simulink model "KUKA_Linear"  (R2020b)
settings: Solver=VariableStepAuto  StartTime=0.0  StopTime=200  RelTol=1e-3
(part 2 of 3)

== matlab function KUKA_Linear/ 4DoF KUKA LWR4+ Dynamics ==
  data: q input; q_dot input; torque input; q_ddot output
function q_ddot = fcn(q,q_dot,torque)
%#codegen

%% parameters
td1 = q_dot(1);
td2 = q_dot(2);
td3 = q_dot(3);
td4 = q_dot(4);

%% Constant

d3 = 0.4;

m1 = 2.7;
m2 = 2.7;
m3 = 2.7;
m4 = 2.7;

cx1 = 0.001340;
cx2 = 0.001340;
cx3 = -0.001340;
cx4 = -0.001340;

cy1 = -0.87777;
cy2 = -0.02622;
cy3 = 0.87777;
cy4 = 0.02622;

cz1 = -0.02622;
cz2 = 0.87777;
cz3 = -0.02622;
cz4 = 0.87777;

g = 9.8;

Ixx1 = 0.039; 
Ixy1 = 3.206e-4;
Ixz1 = 9.415e-5;
Iyy1 = 6.887e-3;
Iyz1 = -2.681e-3;
Izz1 = 0.03698;

Ixx2 = 0.039; 
Ixy2 = 9.415e-5;
Ixz2 = -3.145e-4;
Iyy2 = 0.03698;
Iyz2 = 9.747e-3;
Izz2 = 6.887e-3;

Ixx3 = 6.887e-3; 
Ixy3 = 3.145e-4;
Ixz3 = -9.5572e-5;
Iyy3 = 6.8872e-3;
Iyz3 = 2.681e-3;
Izz3 = 0.037;

Ixx4 = 0.037; 
Ixy4 = 9.415e-5;
Ixz4 = 3.1455e-4;
Iyy4 = 0.037;
Iyz4 = 9.747e-3;
Izz4 = 6.887e-3;

%% Triangle relative
c1 = cos(q(1));
c2 = cos(q(2));
c3 = cos(q(3));
c4 = cos(q(4)); 

s1 = sin(q(1));
s2 = sin(q(2));
s3 = sin(q(3));
s4 = sin(q(4));

%% matrix M

m11 = m1*cx1^2 + m1*cy1^2 + Izz1 - Iyz2*c2 - Ixz2*s2 - s2*(Ixz3*c2 + c3*(Ixx4*(c2*s4 - c3*c4*s2) - Ixy4*(c2*c4 + c3*s2*s4) + cy4*m4*(cy4*(c2*s4 - c3*c4*s2) - cx4*(c2*c4 + c3*s2*s4) + c3*d3*s2) + cz4*m4*(cz4*(c2*s4 - c3*c4*s2) - cx4*s2*s3 + d3*s2*s3*s4) - Ixz4*s2*s3) + s3*(Ixy4*(c2*s4 - c3*c4*s2) - Iyy4*(c2*c4 + c3*s2*s4) + cx4*m4*(cy4*(c2*s4 - c3*c4*s2) - cx4*(c2*c4 + c3*s2*s4) + c3*d3*s2) - cz4*m4*(cz4*(c2*c4 + c3*s2*s4) - cy4*s2*s3 + c4*d3*s2*s3) + Iyz4*s2*s3) - d3*m4*(cy4*(c2*s4 - c3*c4*s2) - cx4*(c2*c4 + c3*s2*s4) + c3*d3*s2) + cz3*m3*(c2*cx3 - c3*cz3*s2) - Ixx3*c3*s2 - Ixy3*s2*s3 - cy3*m3*(c3*cy3*s2 + cx3*s2*s3)) - c2*(Iyz3*c2 + d3*(c3*m4*(cz4*(c2*c4 + c3*s2*s4) - cy4*s2*s3 + c4*d3*s2*s3) + m4*s3*(cz4*(c2*s4 - c3*c4*s2) - cx4*s2*s3 + d3*s2*s3*s4)) - Ixz4*(c2*s4 - c3*c4*s2) - Iyz4*(c2*c4 + c3*s2*s4) - cy4*m4*(cz4*(c2*c4 + c3*s2*s4) - cy4*s2*s3 + c4*d3*s2*s3) - cx4*m4*(cz4*(c2*s4 - c3*c4*s2) - cx4*s2*s3 + d3*s2*s3*s4) + cz3*m3*(c2*cy3 + cz3*s2*s3) + Ixy3*c3*s2 + Iyy3*s2*s3 + Izz4*s2*s3 + cx3*m3*(c3*cy3*s2 + cx3*s2*s3)) - cx2*cz2*m2*s2 - c2*cy2*cz2*m2;
m12 = m2*cx2^2 + m2*cy2^2 + Izz2 - c2*(c3*m3*cz3^2 - d3*(c3*m4*(c3*cy4 - c3*c4*d3 + cz4*s3*s4) - m4*s3*(c4*cz4*s3 - c3*cx4 + c3*d3*s4)) + Iyy3*c3 + Izz4*c3 - Ixy3*s3 - Ixz4*c4*s3 + Iyz4*s3*s4 - cx4*m4*(c4*cz4*s3 - c3*cx4 + c3*d3*s4) + cy4*m4*(c3*cy4 - c3*c4*d3 + cz4*s3*s4) + cx3*m3*(c3*cx3 - cy3*s3)) - s2*(m3*s3*cz3^2 - Ixy3*c3 + Ixx3*s3 + c3*(cy4*m4*(c4*cy4*s3 - d3*s3 + cx4*s3*s4) - Ixz4*c3 + Ixx4*c4*s3 + Ixy4*s3*s4 + cz4*m4*(c4*cz4*s3 - c3*cx4 + c3*d3*s4)) + s3*(Iyz4*c3 + cx4*m4*(c4*cy4*s3 - d3*s3 + cx4*s3*s4) + Ixy4*c4*s3 + Iyy4*s3*s4 + cz4*m4*(c3*cy4 - c3*c4*d3 + cz4*s3*s4)) - d3*m4*(c4*cy4*s3 - d3*s3 + cx4*s3*s4) - cy3*m3*(c3*cx3 - cy3*s3));
m13 = c2*(Iyz4*c4 - Iyz3 + Ixz4*s4 - d3*(cz4*m4*s3*s4 + c3*c4*cz4*m4) - cy3*cz3*m3 + cx4*cz4*m4*s4 + c4*cy4*cz4*m4) - s2*(Ixz3 - c3*(- m4*s4*cz4^2 + Ixy4*c4 - Ixx4*s4 + cy4*m4*(c4*cx4 - cy4*s4)) - s3*(c4*m4*cz4^2 + Iyy4*c4 - Ixy4*s4 + cx4*m4*(c4*cx4 - cy4*s4)) + cx3*cz3*m3 + d3*m4*(c4*cx4 - cy4*s4));
m14 = s2*(s3*(Iyz4 + cy4*cz4*m4) - c3*(Ixz4 + cx4*cz4*m4)) + c2*(Izz4 - d3*(c3*cy4*m4 + cx4*m4*s3) + cx4^2*m4 + cy4^2*m4);

m21 = - Iyz2*c2 - Ixz2*s2 - s2*(Ixz3*c2 + c3*(Ixx4*(c2*s4 - c3*c4*s2) - Ixy4*(c2*c4 + c3*s2*s4) + cy4*m4*(cy4*(c2*s4 - c3*c4*s2) - cx4*(c2*c4 + c3*s2*s4) + c3*d3*s2) + cz4*m4*(cz4*(c2*s4 - c3*c4*s2) - cx4*s2*s3 + d3*s2*s3*s4) - Ixz4*s2*s3) + s3*(Ixy4*(c2*s4 - c3*c4*s2) - Iyy4*(c2*c4 + c3*s2*s4) + cx4*m4*(cy4*(c2*s4 - c3*c4*s2) - cx4*(c2*c4 + c3*s2*s4) + c3*d3*s2) - cz4*m4*(cz4*(c2*c4 + c3*s2*s4) - cy4*s2*s3 + c4*d3*s2*s3) + Iyz4*s2*s3) - d3*m4*(cy4*(c2*s4 - c3*c4*s2) - cx4*(c2*c4 + c3*s2*s4) + c3*d3*s2) + cz3*m3*(c2*cx3 - c3*cz3*s2) - Ixx3*c3*s2 - Ixy3*s2*s3 - cy3*m3*(c3*cy3*s2 + cx3*s2*s3)) - c2*(Iyz3*c2 + d3*(c3*m4*(cz4*(c2*c4 + c3*s2*s4) - cy4*s2*s3 + c4*d3*s2*s3) + m4*s3*(cz4*(c2*s4 - c3*c4*s2) - cx4*s2*s3 + d3*s2*s3*s4)) - Ixz4*(c2*s4 - c3*c4*s2) - Iyz4*(c2*c4 + c3*s2*s4) - cy4*m4*(cz4*(c2*c4 + c3*s2*s4) - cy4*s2*s3 + c4*d3*s2*s3) - cx4*m4*(cz4*(c2*s4 - c3*c4*s2) - cx4*s2*s3 + d3*s2*s3*s4) + cz3*m3*(c2*cy3 + cz3*s2*s3) + Ixy3*c3*s2 + Iyy3*s2*s3 + Izz4*s2*s3 + cx3*m3*(c3*cy3*s2 + cx3*s2*s3)) - cx2*cz2*m2*s2 - c2*cy2*cz2*m2;
m22 = m2*cx2^2 + m2*cy2^2 + Izz2 - c2*(c3*m3*cz3^2 - d3*(c3*m4*(c3*cy4 - c3*c4*d3 + cz4*s3*s4) - m4*s3*(c4*cz4*s3 - c3*cx4 + c3*d3*s4)) + Iyy3*c3 + Izz4*c3 - Ixy3*s3 - Ixz4*c4*s3 + Iyz4*s3*s4 - cx4*m4*(c4*cz4*s3 - c3*cx4 + c3*d3*s4) + cy4*m4*(c3*cy4 - c3*c4*d3 + cz4*s3*s4) + cx3*m3*(c3*cx3 - cy3*s3)) - s2*(m3*s3*cz3^2 - Ixy3*c3 + Ixx3*s3 + c3*(cy4*m4*(c4*cy4*s3 - d3*s3 + cx4*s3*s4) - Ixz4*c3 + Ixx4*c4*s3 + Ixy4*s3*s4 + cz4*m4*(c4*cz4*s3 - c3*cx4 + c3*d3*s4)) + s3*(Iyz4*c3 + cx4*m4*(c4*cy4*s3 - d3*s3 + cx4*s3*s4) + Ixy4*c4*s3 + Iyy4*s3*s4 + cz4*m4*(c3*cy4 - c3*c4*d3 + cz4*s3*s4)) - d3*m4*(c4*cy4*s3 - d3*s3 + cx4*s3*s4) - cy3*m3*(c3*cx3 - cy3*s3));
m23 = c2*(Iyz4*c4 - Iyz3 + Ixz4*s4 - d3*(cz4*m4*s3*s4 + c3*c4*cz4*m4) - cy3*cz3*m3 + cx4*cz4*m4*s4 + c4*cy4*cz4*m4) - s2*(Ixz3 - c3*(- m4*s4*cz4^2 + Ixy4*c4 - Ixx4*s4 + cy4*m4*(c4*cx4 - cy4*s4)) - s3*(c4*m4*cz4^2 + Iyy4*c4 - Ixy4*s4 + cx4*m4*(c4*cx4 - cy4*s4)) + cx3*cz3*m3 + d3*m4*(c4*cx4 - cy4*s4));
m24 = s2*(s3*(Iyz4 + cy4*cz4*m4) - c3*(Ixz4 + cx4*cz4*m4)) + c2*(Izz4 - d3*(c3*cy4*m4 + cx4*m4*s3) + cx4^2*m4 + cy4^2*m4);

m31 = Izz3*c2 - c3*(Ixy4*(c2*s4 - c3*c4*s2) - Iyy4*(c2*c4 + c3*s2*s4) + cx4*m4*(cy4*(c2*s4 - c3*c4*s2) - cx4*(c2*c4 + c3*s2*s4) + c3*d3*s2) - cz4*m4*(cz4*(c2*c4 + c3*s2*s4) - cy4*s2*s3 + c4*d3*s2*s3) + Iyz4*s2*s3) + s3*(Ixx4*(c2*s4 - c3*c4*s2) - Ixy4*(c2*c4 + c3*s2*s4) + cy4*m4*(cy4*(c2*s4 - c3*c4*s2) - cx4*(c2*c4 + c3*s2*s4) + c3*d3*s2) + cz4*m4*(cz4*(c2*s4 - c3*c4*s2) - cx4*s2*s3 + d3*s2*s3*s4) - Ixz4*s2*s3) + cx3*m3*(c2*cx3 - c3*cz3*s2) + cy3*m3*(c2*cy3 + cz3*s2*s3) - Ixz3*c3*s2 + Iyz3*s2*s3;
m32 = Iyz3*c3 + Ixz3*s3 - c3*(Iyz4*c3 + cx4*m4*(c4*cy4*s3 - d3*s3 + cx4*s3*s4) + Ixy4*c4*s3 + Iyy4*s3*s4 + cz4*m4*(c3*cy4 - c3*c4*d3 + cz4*s3*s4)) + s3*(cy4*m4*(c4*cy4*s3 - d3*s3 + cx4*s3*s4) - Ixz4*c3 + Ixx4*c4*s3 + Ixy4*s3*s4 + cz4*m4*(c4*cz4*s3 - c3*cx4 + c3*d3*s4)) + cx3*cz3*m3*s3 + c3*cy3*cz3*m3;
m33 = m3*cx3^2 + m3*cy3^2 + Izz3 + c3*(c4*m4*cz4^2 + Iyy4*c4 - Ixy4*s4 + cx4*m4*(c4*cx4 - cy4*s4)) - s3*(- m4*s4*cz4^2 + Ixy4*c4 - Ixx4*s4 + cy4*m4*(c4*cx4 - cy4*s4));
m34 = s3*(Ixz4 + cx4*cz4*m4) + c3*(Iyz4 + cy4*cz4*m4);

m41 = Ixz4*(c2*s4 - c3*c4*s2) + Iyz4*(c2*c4 + c3*s2*s4) + cy4*m4*(cz4*(c2*c4 + c3*s2*s4) - cy4*s2*s3 + c4*d3*s2*s3) + cx4*m4*(cz4*(c2*s4 - c3*c4*s2) - cx4*s2*s3 + d3*s2*s3*s4) - Izz4*s2*s3;
m42 = Ixz4*c4*s3 - Izz4*c3 - Iyz4*s3*s4 + cx4*m4*(c4*cz4*s3 - c3*cx4 + c3*d3*s4) - cy4*m4*(c3*cy4 - c3*c4*d3 + cz4*s3*s4);
m43 = Iyz4*c4 + Ixz4*s4 + cx4*cz4*m4*s4 + c4*cy4*cz4*m4;
m44 = m4*cx4^2 + m4*cy4^2 + Izz4;

M = [m11 m12 m13 m14;
     m21 m22 m23 m24;
     m31 m32 m33 m34;
     m41 m42 m43 m44];
 
%% matrix V

corio1 = (td2^2*(c2*(2*s3*(Iyz3*c3 + Ixz3*s3) - d3*(c3*m4*(2*c3*(c3*cx4 - c4*cz4*s3) - s4*(2*d3*c3^2 + 2*d3*s3^2) + 2*s3*s4*(c4*cy4*s3 + cx4*s3*s4)) - m4*s3*(2*c3*(c3*cy4 + cz4*s3*s4) - c4*(2*d3*c3^2 + 2*d3*s3^2) + 2*c4*s3*(c4*cy4*s3 + cx4*s3*s4))) - cx4*m4*(2*c3*(c3*cy4 + cz4*s3*s4) - c4*(2*d3*c3^2 + 2*d3*s3^2) + 2*c4*s3*(c4*cy4*s3 + cx4*s3*s4)) + cy4*m4*(2*c3*(c3*cx4 - c4*cz4*s3) - s4*(2*d3*c3^2 + 2*d3*s3^2) + 2*s3*s4*(c4*cy4*s3 + cx4*s3*s4)) + cx3*m3*(2*cz3*c3^2 + 2*cz3*s3^2) - 2*c4*s3*(Iyz4*c3 + Ixy4*c4*s3 + Iyy4*s3*s4) + 2*s3*s4*(Ixx4*c4*s3 - Ixz4*c3 + Ixy4*s3*s4) - 2*c3*cz3*m3*(c3*cx3 - cy3*s3)) - s2*(2*c3*(Iyz3*c3 + Ixz3*s3) - s3*(cx4*m4*(2*c4*s3*(c3*cx4 - c4*cz4*s3) - 2*s3*s4*(c3*cy4 + cz4*s3*s4)) - 2*c3*(Ixx4*c4*s3 - Ixz4*c3 + Ixy4*s3*s4) + cz4*m4*(2*c3*(c3*cx4 - c4*cz4*s3) - s4*(2*d3*c3^2 + 2*d3*s3^2) + 2*s3*s4*(c4*cy4*s3 + cx4*s3*s4)) + 2*c4*s3*(Izz4*c3 - Ixz4*c4*s3 + Iyz4*s3*s4)) - c3*(2*c3*(Iyz4*c3 + Ixy4*c4*s3 + Iyy4*s3*s4) + cy4*m4*(2*c4*s3*(c3*cx4 - c4*cz4*s3) - 2*s3*s4*(c3*cy4 + cz4*s3*s4)) + cz4*m4*(2*c3*(c3*cy4 + cz4*s3*s4) - c4*(2*d3*c3^2 + 2*d3*s3^2) + 2*c4*s3*(c4*cy4*s3 + cx4*s3*s4)) - 2*s3*s4*(Izz4*c3 - Ixz4*c4*s3 + Iyz4*s3*s4)) + d3*m4*(2*c4*s3*(c3*cx4 - c4*cz4*s3) - 2*s3*s4*(c3*cy4 + cz4*s3*s4)) + cy3*m3*(2*cz3*c3^2 + 2*cz3*s3^2) + 2*cz3*m3*s3*(c3*cx3 - cy3*s3))))/2 + (td3^2*(s2*(2*Iyz3 - c3*(2*c4*(Iyz4*c4 + Ixz4*s4) + cy4*m4*(2*cz4*c4^2 + 2*cz4*s4^2) + 2*cz4*m4*s4*(c4*cx4 - cy4*s4)) - s3*(2*s4*(Iyz4*c4 + Ixz4*s4) + cx4*m4*(2*cz4*c4^2 + 2*cz4*s4^2) - 2*c4*cz4*m4*(c4*cx4 - cy4*s4)) + 2*cy3*cz3*m3 + d3*m4*(2*cz4*c4^2 + 2*cz4*s4^2)) + c2*(2*c4*(Ixy4*c4 - Ixx4*s4) - 2*Ixz3 + 2*s4*(Iyy4*c4 - Ixy4*s4) - d3*(2*c3*c4*m4*(c4*cx4 - cy4*s4) + 2*m4*s3*s4*(c4*cx4 - cy4*s4)) - 2*cx3*cz3*m3 + 2*c4*cy4*m4*(c4*cx4 - cy4*s4) + 2*cx4*m4*s4*(c4*cx4 - cy4*s4))))/2 + (td4^2*(s2*(c3*(2*Iyz4 + 2*cy4*cz4*m4) + s3*(2*Ixz4 + 2*cx4*cz4*m4)) - c2*d3*(2*c3*cx4*m4 - 2*cy4*m4*s3)))/2 + (td1^2*(s2*(2*c2*(Iyz3*c2 + Ixy3*c3*s2 + Iyy3*s2*s3) - c3*(2*(c2*c4 + c3*s2*s4)*(Ixz4*(c2*s4 - c3*c4*s2) + Iyz4*(c2*c4 + c3*s2*s4) - Izz4*s2*s3) + cy4*m4*(2*(c2*s4 - c3*c4*s2)*(cz4*(c2*s4 - c3*c4*s2) - cx4*s2*s3) + 2*(c2*c4 + c3*s2*s4)*(cz4*(c2*c4 + c3*s2*s4) - cy4*s2*s3) + 2*c2*d3*s2*s3) - 2*s2*s3*(Ixy4*(c2*s4 - c3*c4*s2) - Iyy4*(c2*c4 + c3*s2*s4) + Iyz4*s2*s3) + cz4*m4*(2*(c2*s4 - c3*c4*s2)*(cx4*(c2*c4 + c3*s2*s4) - cy4*(c2*s4 - c3*c4*s2)) + c4*(2*d3*c3^2*s2^2 + 2*d3*s2^2*s3^2) + 2*s2*s3*(cz4*(c2*c4 + c3*s2*s4) - cy4*s2*s3) - 2*c2*c3*d3*s2*s4)) - s3*(2*(c2*s4 - c3*c4*s2)*(Ixz4*(c2*s4 - c3*c4*s2) + Iyz4*(c2*c4 + c3*s2*s4) - Izz4*s2*s3) + cx4*m4*(2*(c2*s4 - c3*c4*s2)*(cz4*(c2*s4 - c3*c4*s2) - cx4*s2*s3) + 2*(c2*c4 + c3*s2*s4)*(cz4*(c2*c4 + c3*s2*s4) - cy4*s2*s3) + 2*c2*d3*s2*s3) - 2*s2*s3*(Ixy4*(c2*c4 + c3*s2*s4) - Ixx4*(c2*s4 - c3*c4*s2) + Ixz4*s2*s3) + cz4*m4*(s4*(2*d3*c3^2*s2^2 + 2*d3*s2^2*s3^2) - 2*(c2*c4 + c3*s2*s4)*(cx4*(c2*c4 + c3*s2*s4) - cy4*(c2*s4 - c3*c4*s2)) + 2*s2*s3*(cz4*(c2*s4 - c3*c4*s2) - cx4*s2*s3) + 2*c2*c3*c4*d3*s2)) + cz3*m3*(2*c2*(c2*cy3 + cz3*s2*s3) + 2*c3*s2*(c3*cy3*s2 + cx3*s2*s3)) + cy3*m3*(2*c3*s2*(c2*cx3 - c3*cz3*s2) - 2*s2*s3*(c2*cy3 + cz3*s2*s3)) + d3*m4*(2*(c2*s4 - c3*c4*s2)*(cz4*(c2*s4 - c3*c4*s2) - cx4*s2*s3) + 2*(c2*c4 + c3*s2*s4)*(cz4*(c2*c4 + c3*s2*s4) - cy4*s2*s3) + 2*c2*d3*s2*s3) - 2*s2*s3*(Izz3*c2 - Ixz3*c3*s2 + Iyz3*s2*s3)) + 2*c2*(Ixy2*c2 - Ixx2*s2) + 2*s2*(Iyy2*c2 - Ixy2*s2) - c2*(2*(c2*s4 - c3*c4*s2)*(Ixy4*(c2*s4 - c3*c4*s2) - Iyy4*(c2*c4 + c3*s2*s4) + Iyz4*s2*s3) - 2*(c2*c4 + c3*s2*s4)*(Ixy4*(c2*c4 + c3*s2*s4) - Ixx4*(c2*s4 - c3*c4*s2) + Ixz4*s2*s3) - d3*(c3*m4*(s4*(2*d3*c3^2*s2^2 + 2*d3*s2^2*s3^2) - 2*(c2*c4 + c3*s2*s4)*(cx4*(c2*c4 + c3*s2*s4) - cy4*(c2*s4 - c3*c4*s2)) + 2*s2*s3*(cz4*(c2*s4 - c3*c4*s2) - cx4*s2*s3) + 2*c2*c3*c4*d3*s2) - m4*s3*(2*(c2*s4 - c3*c4*s2)*(cx4*(c2*c4 + c3*s2*s4) - cy4*(c2*s4 - c3*c4*s2)) + c4*(2*d3*c3^2*s2^2 + 2*d3*s2^2*s3^2) + 2*s2*s3*(cz4*(c2*c4 + c3*s2*s4) - cy4*s2*s3) - 2*c2*c3*d3*s2*s4)) - 2*c2*(Ixx3*c3*s2 - Ixz3*c2 + Ixy3*s2*s3) + cx3*m3*(2*c3*s2*(c2*cx3 - c3*cz3*s2) - 2*s2*s3*(c2*cy3 + cz3*s2*s3)) + cz3*m3*(2*c2*(c2*cx3 - c3*cz3*s2) + 2*s2*s3*(c3*cy3*s2 + cx3*s2*s3)) + 2*c3*s2*(Izz3*c2 - Ixz3*c3*s2 + Iyz3*s2*s3) - cx4*m4*(2*(c2*s4 - c3*c4*s2)*(cx4*(c2*c4 + c3*s2*s4) - cy4*(c2*s4 - c3*c4*s2)) + c4*(2*d3*c3^2*s2^2 + 2*d3*s2^2*s3^2) + 2*s2*s3*(cz4*(c2*c4 + c3*s2*s4) - cy4*s2*s3) - 2*c2*c3*d3*s2*s4) + cy4*m4*(s4*(2*d3*c3^2*s2^2 + 2*d3*s2^2*s3^2) - 2*(c2*c4 + c3*s2*s4)*(cx4*(c2*c4 + c3*s2*s4) - cy4*(c2*s4 - c3*c4*s2)) + 2*s2*s3*(cz4*(c2*s4 - c3*c4*s2) - cx4*s2*s3) + 2*c2*c3*c4*d3*s2)) + 2*c2*cy2*m2*(c2*cx2 - cy2*s2) + 2*cx2*m2*s2*(c2*cx2 - cy2*s2)))/2 - td2*td4*(s2*(s3*(2*Ixz4*c3 - Ixx4*c4*s3 + Iyy4*c4*s3 + Izz4*c4*s3 - 2*Ixy4*s3*s4 + cx4*m4*(2*c4*cx4*s3 - 2*cy4*s3*s4) + 2*c3*cx4*cz4*m4) + c3*(2*Iyz4*c3 + 2*Ixy4*c4*s3 - Ixx4*s3*s4 + Iyy4*s3*s4 - Izz4*s3*s4 + cy4*m4*(2*c4*cx4*s3 - 2*cy4*s3*s4) + 2*c3*cy4*cz4*m4) - d3*m4*(2*c4*cx4*s3 - 2*cy4*s3*s4)) - c2*d3*(2*c3^2*cx4*m4 - 2*c3*cy4*m4*s3)) - td1*td3*(c2*(2*Ixz3*c2 - (c2*c4 + c3*s2*s4)*(Ixy4*c4 - Ixx4*s4) - (c2*s4 - c3*c4*s2)*(Iyy4*c4 - Ixy4*s4) + d3*(c3*m4*(c4*(cx4*(c2*c4 + c3*s2*s4) - cy4*(c2*s4 - c3*c4*s2)) + (c2*c4 + c3*s2*s4)*(c4*cx4 - cy4*s4) - c3*cy4*s2 - 2*cz4*s2*s3*s4) + m4*s3*(s4*(cx4*(c2*c4 + c3*s2*s4) - cy4*(c2*s4 - c3*c4*s2)) + (c2*s4 - c3*c4*s2)*(c4*cx4 - cy4*s4) - c3*cx4*s2 + 2*c4*cz4*s2*s3)) - c4*(Ixy4*(c2*c4 + c3*s2*s4) - Ixx4*(c2*s4 - c3*c4*s2) + Ixz4*s2*s3) + s4*(Ixy4*(c2*s4 - c3*c4*s2) - Iyy4*(c2*c4 + c3*s2*s4) + Iyz4*s2*s3) - Ixx3*c3*s2 + Iyy3*c3*s2 + Izz3*c3*s2 + Izz4*c3*s2 - cx4*m4*(s4*(cx4*(c2*c4 + c3*s2*s4) - cy4*(c2*s4 - c3*c4*s2)) + (c2*s4 - c3*c4*s2)*(c4*cx4 - cy4*s4) - c3*cx4*s2 + 2*c4*cz4*s2*s3) - cy4*m4*(c4*(cx4*(c2*c4 + c3*s2*s4) - cy4*(c2*s4 - c3*c4*s2)) + (c2*c4 + c3*s2*s4)*(c4*cx4 - cy4*s4) - c3*cy4*s2 - 2*cz4*s2*s3*s4) - 2*Ixy3*s2*s3 + cx3*m3*(2*c3*cx3*s2 - 2*cy3*s2*s3) + Iyz4*s2*s3*s4 - Ixz4*c4*s2*s3 + 2*c2*cx3*cz3*m3) - s2*(2*Iyz3*c2 - c3*((c2*c4 + c3*s2*s4)*(Iyz4*c4 + Ixz4*s4) + c4*(Ixz4*(c2*s4 - c3*c4*s2) + Iyz4*(c2*c4 + c3*s2*s4) - Izz4*s2*s3) - Ixz4*c3*s2 + cz4*m4*(s4*(cx4*(c2*c4 + c3*s2*s4) - cy4*(c2*s4 - c3*c4*s2)) + (c2*s4 - c3*c4*s2)*(c4*cx4 - cy4*s4) - c3*cx4*s2 + 2*c4*cz4*s2*s3) + s2*s3*(Iyy4*c4 - Ixy4*s4) + cy4*m4*(c4*(cz4*(c2*c4 + c3*s2*s4) - cy4*s2*s3) + s4*(cz4*(c2*s4 - c3*c4*s2) - cx4*s2*s3) + c4*cz4*(c2*c4 + c3*s2*s4) + cz4*s4*(c2*s4 - c3*c4*s2) + c4*cy4*s2*s3 + cx4*s2*s3*s4) + Ixy4*s2*s3*s4 + Ixx4*c4*s2*s3) - s3*((c2*s4 - c3*c4*s2)*(Iyz4*c4 + Ixz4*s4) + s4*(Ixz4*(c2*s4 - c3*c4*s2) + Iyz4*(c2*c4 + c3*s2*s4) - Izz4*s2*s3) + Iyz4*c3*s2 - cz4*m4*(c4*(cx4*(c2*c4 + c3*s2*s4) - cy4*(c2*s4 - c3*c4*s2)) + (c2*c4 + c3*s2*s4)*(c4*cx4 - cy4*s4) - c3*cy4*s2 - 2*cz4*s2*s3*s4) - s2*s3*(Ixy4*c4 - Ixx4*s4) + cx4*m4*(c4*(cz4*(c2*c4 + c3*s2*s4) - cy4*s2*s3) + s4*(cz4*(c2*s4 - c3*c4*s2) - cx4*s2*s3) + c4*cz4*(c2*c4 + c3*s2*s4) + cz4*s4*(c2*s4 - c3*c4*s2) + c4*cy4*s2*s3 + cx4*s2*s3*s4) + Iyy4*s2*s3*s4 + Ixy4*c4*s2*s3) + 2*Ixy3*c3*s2 - Ixx3*s2*s3 + Iyy3*s2*s3 - Izz3*s2*s3 + cy3*m3*(2*c3*cx3*s2 - 2*cy3*s2*s3) + d3*m4*(c4*(cz4*(c2*c4 + c3*s2*s4) - cy4*s2*s3) + s4*(cz4*(c2*s4 - c3*c4*s2) - cx4*s2*s3) + c4*cz4*(c2*c4 + c3*s2*s4) + cz4*s4*(c2*s4 - c3*c4*s2) + c4*cy4*s2*s3 + cx4*s2*s3*s4) + 2*c2*cy3*cz3*m3)) - td1*td4*(s2*(s3*(2*Ixy4*(c2*c4 + c3*s2*s4) - Ixx4*(c2*s4 - c3*c4*s2) + Iyy4*(c2*s4 - c3*c4*s2) + Izz4*(c2*s4 - c3*c4*s2) + cx4*m4*(2*cx4*(c2*s4 - c3*c4*s2) + 2*cy4*(c2*c4 + c3*s2*s4)) + 2*Ixz4*s2*s3 + 2*cx4*cz4*m4*s2*s3) + c3*(Ixx4*(c2*c4 + c3*s2*s4) + 2*Ixy4*(c2*s4 - c3*c4*s2) - Iyy4*(c2*c4 + c3*s2*s4) + Izz4*(c2*c4 + c3*s2*s4) + cy4*m4*(2*cx4*(c2*s4 - c3*c4*s2) + 2*cy4*(c2*c4 + c3*s2*s4)) + 2*Iyz4*s2*s3 + 2*cy4*cz4*m4*s2*s3) - d3*m4*(2*cx4*(c2*s4 - c3*c4*s2) + 2*cy4*(c2*c4 + c3*s2*s4))) + c2*d3*(2*cy4*m4*s2*s3^2 - 2*c3*cx4*m4*s2*s3)) - td2*td3*(s2*(Ixx3*c3 - Iyy3*c3 + Izz3*c3 + 2*Ixy3*s3 + c3*(Ixz4*s3 - c4*(Izz4*c3 - Ixz4*c4*s3 + Iyz4*s3*s4) + c3*(Iyy4*c4 - Ixy4*s4) + Ixx4*c3*c4 + Ixy4*c3*s4 - cy4*m4*(s4*(c3*cx4 - c4*cz4*s3) + c4*(c3*cy4 + cz4*s3*s4) - c3*c4*cy4 - c3*cx4*s4) + cz4*m4*(cx4*s3 - s4*(c4*cy4*s3 + cx4*s3*s4) + 2*c3*c4*cz4 + c4*s3*(c4*cx4 - cy4*s4)) - s3*s4*(Iyz4*c4 + Ixz4*s4)) - s3*(Iyz4*s3 + c3*(Ixy4*c4 - Ixx4*s4) + s4*(Izz4*c3 - Ixz4*c4*s3 + Iyz4*s3*s4) - Ixy4*c3*c4 - Iyy4*c3*s4 + cx4*m4*(s4*(c3*cx4 - c4*cz4*s3) + c4*(c3*cy4 + cz4*s3*s4) - c3*c4*cy4 - c3*cx4*s4) - c4*s3*(Iyz4*c4 + Ixz4*s4) - cz4*m4*(c4*(c4*cy4*s3 + cx4*s3*s4) - cy4*s3 + s3*s4*(c4*cx4 - cy4*s4) + 2*c3*cz4*s4)) + d3*m4*(s4*(c3*cx4 - c4*cz4*s3) + c4*(c3*cy4 + cz4*s3*s4) - c3*c4*cy4 - c3*cx4*s4) + cy3*m3*(2*c3*cy3 + 2*cx3*s3)) - c2*(2*Ixy3*c3 - Ixx3*s3 + Iyy3*s3 + Izz3*s3 + Izz4*s3 - c4*(Ixx4*c4*s3 - Ixz4*c3 + Ixy4*s3*s4) - s4*(Iyz4*c3 + Ixy4*c4*s3 + Iyy4*s3*s4) - d3*(m4*s3*(cx4*s3 - s4*(c4*cy4*s3 + cx4*s3*s4) + 2*c3*c4*cz4 + c4*s3*(c4*cx4 - cy4*s4)) - c3*m4*(c4*(c4*cy4*s3 + cx4*s3*s4) - cy4*s3 + s3*s4*(c4*cx4 - cy4*s4) + 2*c3*cz4*s4)) + Ixz4*c3*c4 - Iyz4*c3*s4 + cx4*m4*(cx4*s3 - s4*(c4*cy4*s3 + cx4*s3*s4) + 2*c3*c4*cz4 + c4*s3*(c4*cx4 - cy4*s4)) + c4*s3*(Iyy4*c4 - Ixy4*s4) - cy4*m4*(c4*(c4*cy4*s3 + cx4*s3*s4) - cy4*s3 + s3*s4*(c4*cx4 - cy4*s4) + 2*c3*cz4*s4) - s3*s4*(Ixy4*c4 - Ixx4*s4) + cx3*m3*(2*c3*cy3 + 2*cx3*s3))) - td1*td2*(c2*((c2*c4 + c3*s2*s4)*(Ixx4*c4*s3 - Ixz4*c3 + Ixy4*s3*s4) + (c2*s4 - c3*c4*s2)*(Iyz4*c3 + Ixy4*c4*s3 + Iyy4*s3*s4) - d3*(m4*s3*((c2*s4 - c3*c4*s2)*(c4*cy4*s3 + cx4*s3*s4) - c3*(cz4*(c2*c4 + c3*s2*s4) - cy4*s2*s3) + cz4*(s2*s4 + c2*c3*c4) + s2*s3*(c3*cy4 + cz4*s3*s4) - c4*s3*(cx4*(c2*c4 + c3*s2*s4) - cy4*(c2*s4 - c3*c4*s2)) + c2*cx4*s3 - 2*c2*d3*s3*s4) + c3*m4*((c2*c4 + c3*s2*s4)*(c4*cy4*s3 + cx4*s3*s4) + c3*(cz4*(c2*s4 - c3*c4*s2) - cx4*s2*s3) + cz4*(c4*s2 - c2*c3*s4) - s2*s3*(c3*cx4 - c4*cz4*s3) + s3*s4*(cx4*(c2*c4 + c3*s2*s4) - cy4*(c2*s4 - c3*c4*s2)) + c2*cy4*s3 - 2*c2*c4*d3*s3)) - Iyz3*s2 - c2*(Ixy3*c3 - Ixx3*s3) - s3*(Izz3*c2 - Ixz3*c3*s2 + Iyz3*s2*s3) + Ixz4*(s2*s4 + c2*c3*c4) + Iyz4*(c4*s2 - c2*c3*s4) + Ixy3*c2*c3 + Iyy3*c2*s3 + Izz4*c2*s3 - cx3*m3*(s3*(c2*cx3 - c3*cz3*s2) + c3*(c2*cy3 + cz3*s2*s3) - c2*c3*cy3 - c2*cx3*s3) + c3*s2*(Iyz3*c3 + Ixz3*s3) + cz3*m3*(c3*(c3*cy3*s2 + cx3*s2*s3) - cy3*s2 + s2*s3*(c3*cx3 - cy3*s3) + 2*c2*cz3*s3) + c4*s3*(Ixy4*(c2*s4 - c3*c4*s2) - Iyy4*(c2*c4 + c3*s2*s4) + Iyz4*s2*s3) + s3*s4*(Ixy4*(c2*c4 + c3*s2*s4) - Ixx4*(c2*s4 - c3*c4*s2) + Ixz4*s2*s3) + cy4*m4*((c2*c4 + c3*s2*s4)*(c4*cy4*s3 + cx4*s3*s4) + c3*(cz4*(c2*s4 - c3*c4*s2) - cx4*s2*s3) + cz4*(c4*s2 - c2*c3*s4) - s2*s3*(c3*cx4 - c4*cz4*s3) + s3*s4*(cx4*(c2*c4 + c3*s2*s4) - cy4*(c2*s4 - c3*c4*s2)) + c2*cy4*s3 - 2*c2*c4*d3*s3) + cx4*m4*((c2*s4 - c3*c4*s2)*(c4*cy4*s3 + cx4*s3*s4) - c3*(cz4*(c2*c4 + c3*s2*s4) - cy4*s2*s3) + cz4*(s2*s4 + c2*c3*c4) + s2*s3*(c3*cy4 + cz4*s3*s4) - c4*s3*(cx4*(c2*c4 + c3*s2*s4) - cy4*(c2*s4 - c3*c4*s2)) + c2*cx4*s3 - 2*c2*d3*s3*s4)) - s2*(c3*((c2*c4 + c3*s2*s4)*(Izz4*c3 - Ixz4*c4*s3 + Iyz4*s3*s4) + c3*(Ixy4*(c2*s4 - c3*c4*s2) - Iyy4*(c2*c4 + c3*s2*s4) + Iyz4*s2*s3) + Ixx4*(s2*s4 + c2*c3*c4) - Ixy4*(c4*s2 - c2*c3*s4) + Ixz4*c2*s3 + s2*s3*(Iyz4*c3 + Ixy4*c4*s3 + Iyy4*s3*s4) + cy4*m4*((c3*cx4 - c4*cz4*s3)*(c2*s4 - c3*c4*s2) + (c2*c4 + c3*s2*s4)*(c3*cy4 + cz4*s3*s4) - cx4*(c4*s2 - c2*c3*s4) + cy4*(s2*s4 + c2*c3*c4) - c4*s3*(cz4*(c2*s4 - c3*c4*s2) - cx4*s2*s3) + s3*s4*(cz4*(c2*c4 + c3*s2*s4) - cy4*s2*s3) - 2*c2*c3*d3) + s3*s4*(Ixz4*(c2*s4 - c3*c4*s2) + Iyz4*(c2*c4 + c3*s2*s4) - Izz4*s2*s3) + cz4*m4*((c2*s4 - c3*c4*s2)*(c4*cy4*s3 + cx4*s3*s4) - c3*(cz4*(c2*c4 + c3*s2*s4) - cy4*s2*s3) + cz4*(s2*s4 + c2*c3*c4) + s2*s3*(c3*cy4 + cz4*s3*s4) - c4*s3*(cx4*(c2*c4 + c3*s2*s4) - cy4*(c2*s4 - c3*c4*s2)) + c2*cx4*s3 - 2*c2*d3*s3*s4)) - s3*(Iyy4*(c4*s2 - c2*c3*s4) - c3*(Ixy4*(c2*c4 + c3*s2*s4) - Ixx4*(c2*s4 - c3*c4*s2) + Ixz4*s2*s3) - Ixy4*(s2*s4 + c2*c3*c4) - (c2*s4 - c3*c4*s2)*(Izz4*c3 - Ixz4*c4*s3 + Iyz4*s3*s4) + Iyz4*c2*s3 + s2*s3*(Ixx4*c4*s3 - Ixz4*c3 + Ixy4*s3*s4) - cx4*m4*((c3*cx4 - c4*cz4*s3)*(c2*s4 - c3*c4*s2) + (c2*c4 + c3*s2*s4)*(c3*cy4 + cz4*s3*s4) - cx4*(c4*s2 - c2*c3*s4) + cy4*(s2*s4 + c2*c3*c4) - c4*s3*(cz4*(c2*s4 - c3*c4*s2) - cx4*s2*s3) + s3*s4*(cz4*(c2*c4 + c3*s2*s4) - cy4*s2*s3) - 2*c2*c3*d3) + c4*s3*(Ixz4*(c2*s4 - c3*c4*s2) + Iyz4*(c2*c4 + c3*s2*s4) - Izz4*s2*s3) + cz4*m4*((c2*c4 + c3*s2*s4)*(c4*cy4*s3 + cx4*s3*s4) + c3*(cz4*(c2*s4 - c3*c4*s2) - cx4*s2*s3) + cz4*(c4*s2 - c2*c3*s4) - s2*s3*(c3*cx4 - c4*cz4*s3) + s3*s4*(cx4*(c2*c4 + c3*s2*s4) - cy4*(c2*s4 - c3*c4*s2)) + c2*cy4*s3 - 2*c2*c4*d3*s3)) + Ixz3*s2 - c3*(Izz3*c2 - Ixz3*c3*s2 + Iyz3*s2*s3) + c2*(Iyy3*c3 - Ixy3*s3) + Ixx3*c2*c3 + Ixy3*c2*s3 - cy3*m3*(s3*(c2*cx3 - c3*cz3*s2) + c3*(c2*cy3 + cz3*s2*s3) - c2*c3*cy3 - c2*cx3*s3) + cz3*m3*(cx3*s2 - s3*(c3*cy3*s2 + cx3*s2*s3) + 2*c2*c3*cz3 + c3*s2*(c3*cx3 - cy3*s3)) - d3*m4*((c3*cx4 - c4*cz4*s3)*(c2*s4 - c3*c4*s2) + (c2*c4 + c3*s2*s4)*(c3*cy4 + cz4*s3*s4) - cx4*(c4*s2 - c2*c3*s4) + cy4*(s2*s4 + c2*c3*c4) - c4*s3*(cz4*(c2*s4 - c3*c4*s2) - cx4*s2*s3) + s3*s4*(cz4*(c2*c4 + c3*s2*s4) - cy4*s2*s3) - 2*c2*c3*d3) - s2*s3*(Iyz3*c3 + Ixz3*s3))) - s2*td3*td4*(c3*(Ixx4*c4 - Iyy4*c4 + Izz4*c4 + 2*Ixy4*s4 + cy4*m4*(2*c4*cy4 + 2*cx4*s4)) + s3*(2*Ixy4*c4 - Ixx4*s4 + Iyy4*s4 + Izz4*s4 + cx4*m4*(2*c4*cy4 + 2*cx4*s4)) - d3*m4*(2*c4*cy4 + 2*cx4*s4));
corio2 = (td2^2*(c2*(2*s3*(Iyz3*c3 + Ixz3*s3) - d3*(c3*m4*(2*c3*(c3*cx4 - c4*cz4*s3) - s4*(2*d3*c3^2 + 2*d3*s3^2) + 2*s3*s4*(c4*cy4*s3 + cx4*s3*s4)) - m4*s3*(2*c3*(c3*cy4 + cz4*s3*s4) - c4*(2*d3*c3^2 + 2*d3*s3^2) + 2*c4*s3*(c4*cy4*s3 + cx4*s3*s4))) - cx4*m4*(2*c3*(c3*cy4 + cz4*s3*s4) - c4*(2*d3*c3^2 + 2*d3*s3^2) + 2*c4*s3*(c4*cy4*s3 + cx4*s3*s4)) + cy4*m4*(2*c3*(c3*cx4 - c4*cz4*s3) - s4*(2*d3*c3^2 + 2*d3*s3^2) + 2*s3*s4*(c4*cy4*s3 + cx4*s3*s4)) + cx3*m3*(2*cz3*c3^2 + 2*cz3*s3^2) - 2*c4*s3*(Iyz4*c3 + Ixy4*c4*s3 + Iyy4*s3*s4) + 2*s3*s4*(Ixx4*c4*s3 - Ixz4*c3 + Ixy4*s3*s4) - 2*c3*cz3*m3*(c3*cx3 - cy3*s3)) - s2*(2*c3*(Iyz3*c3 + Ixz3*s3) - s3*(cx4*m4*(2*c4*s3*(c3*cx4 - c4*cz4*s3) - 2*s3*s4*(c3*cy4 + cz4*s3*s4)) - 2*c3*(Ixx4*c4*s3 - Ixz4*c3 + Ixy4*s3*s4) + cz4*m4*(2*c3*(c3*cx4 - c4*cz4*s3) - s4*(2*d3*c3^2 + 2*d3*s3^2) + 2*s3*s4*(c4*cy4*s3 + cx4*s3*s4)) + 2*c4*s3*(Izz4*c3 - Ixz4*c4*s3 + Iyz4*s3*s4)) - c3*(2*c3*(Iyz4*c3 + Ixy4*c4*s3 + Iyy4*s3*s4) + cy4*m4*(2*c4*s3*(c3*cx4 - c4*cz4*s3) - 2*s3*s4*(c3*cy4 + cz4*s3*s4)) + cz4*m4*(2*c3*(c3*cy4 + cz4*s3*s4) - c4*(2*d3*c3^2 + 2*d3*s3^2) + 2*c4*s3*(c4*cy4*s3 + cx4*s3*s4)) - 2*s3*s4*(Izz4*c3 - Ixz4*c4*s3 + Iyz4*s3*s4)) + d3*m4*(2*c4*s3*(c3*cx4 - c4*cz4*s3) - 2*s3*s4*(c3*cy4 + cz4*s3*s4)) + cy3*m3*(2*cz3*c3^2 + 2*cz3*s3^2) + 2*cz3*m3*s3*(c3*cx3 - cy3*s3))))/2 + (td3^2*(s2*(2*Iyz3 - c3*(2*c4*(Iyz4*c4 + Ixz4*s4) + cy4*m4*(2*cz4*c4^2 + 2*cz4*s4^2) + 2*cz4*m4*s4*(c4*cx4 - cy4*s4)) - s3*(2*s4*(Iyz4*c4 + Ixz4*s4) + cx4*m4*(2*cz4*c4^2 + 2*cz4*s4^2) - 2*c4*cz4*m4*(c4*cx4 - cy4*s4)) + 2*cy3*cz3*m3 + d3*m4*(2*cz4*c4^2 + 2*cz4*s4^2)) + c2*(2*c4*(Ixy4*c4 - Ixx4*s4) - 2*Ixz3 + 2*s4*(Iyy4*c4 - Ixy4*s4) - d3*(2*c3*c4*m4*(c4*cx4 - cy4*s4) + 2*m4*s3*s4*(c4*cx4 - cy4*s4)) - 2*cx3*cz3*m3 + 2*c4*cy4*m4*(c4*cx4 - cy4*s4) + 2*cx4*m4*s4*(c4*cx4 - cy4*s4))))/2 + (td4^2*(s2*(c3*(2*Iyz4 + 2*cy4*cz4*m4) + s3*(2*Ixz4 + 2*cx4*cz4*m4)) - c2*d3*(2*c3*cx4*m4 - 2*cy4*m4*s3)))/2 + (td1^2*(s2*(2*c2*(Iyz3*c2 + Ixy3*c3*s2 + Iyy3*s2*s3) - c3*(2*(c2*c4 + c3*s2*s4)*(Ixz4*(c2*s4 - c3*c4*s2) + Iyz4*(c2*c4 + c3*s2*s4) - Izz4*s2*s3) + cy4*m4*(2*(c2*s4 - c3*c4*s2)*(cz4*(c2*s4 - c3*c4*s2) - cx4*s2*s3) + 2*(c2*c4 + c3*s2*s4)*(cz4*(c2*c4 + c3*s2*s4) - cy4*s2*s3) + 2*c2*d3*s2*s3) - 2*s2*s3*(Ixy4*(c2*s4 - c3*c4*s2) - Iyy4*(c2*c4 + c3*s2*s4) + Iyz4*s2*s3) + cz4*m4*(2*(c2*s4 - c3*c4*s2)*(cx4*(c2*c4 + c3*s2*s4) - cy4*(c2*s4 - c3*c4*s2)) + c4*(2*d3*c3^2*s2^2 + 2*d3*s2^2*s3^2) + 2*s2*s3*(cz4*(c2*c4 + c3*s2*s4) - cy4*s2*s3) - 2*c2*c3*d3*s2*s4)) - s3*(2*(c2*s4 - c3*c4*s2)*(Ixz4*(c2*s4 - c3*c4*s2) + Iyz4*(c2*c4 + c3*s2*s4) - Izz4*s2*s3) + cx4*m4*(2*(c2*s4 - c3*c4*s2)*(cz4*(c2*s4 - c3*c4*s2) - cx4*s2*s3) + 2*(c2*c4 + c3*s2*s4)*(cz4*(c2*c4 + c3*s2*s4) - cy4*s2*s3) + 2*c2*d3*s2*s3) - 2*s2*s3*(Ixy4*(c2*c4 + c3*s2*s4) - Ixx4*(c2*s4 - c3*c4*s2) + Ixz4*s2*s3) + cz4*m4*(s4*(2*d3*c3^2*s2^2 + 2*d3*s2^2*s3^2) - 2*(c2*c4 + c3*s2*s4)*(cx4*(c2*c4 + c3*s2*s4) - cy4*(c2*s4 - c3*c4*s2)) + 2*s2*s3*(cz4*(c2*s4 - c3*c4*s2) - cx4*s2*s3) + 2*c2*c3*c4*d3*s2)) + cz3*m3*(2*c2*(c2*cy3 + cz3*s2*s3) + 2*c3*s2*(c3*cy3*s2 + cx3*s2*s3)) + cy3*m3*(2*c3*s2*(c2*cx3 - c3*cz3*s2) - 2*s2*s3*(c2*cy3 + cz3*s2*s3)) + d3*m4*(2*(c2*s4 - c3*c4*s2)*(cz4*(c2*s4 - c3*c4*s2) - cx4*s2*s3) + 2*(c2*c4 + c3*s2*s4)*(cz4*(c2*c4 + c3*s2*s4) - cy4*s2*s3) + 2*c2*d3*s2*s3) - 2*s2*s3*(Izz3*c2 - Ixz3*c3*s2 + Iyz3*s2*s3)) + 2*c2*(Ixy2*c2 - Ixx2*s2) + 2*s2*(Iyy2*c2 - Ixy2*s2) - c2*(2*(c2*s4 - c3*c4*s2)*(Ixy4*(c2*s4 - c3*c4*s2) - Iyy4*(c2*c4 + c3*s2*s4) + Iyz4*s2*s3) - 2*(c2*c4 + c3*s2*s4)*(Ixy4*(c2*c4 + c3*s2*s4) - Ixx4*(c2*s4 - c3*c4*s2) + Ixz4*s2*s3) - d3*(c3*m4*(s4*(2*d3*c3^2*s2^2 + 2*d3*s2^2*s3^2) - 2*(c2*c4 + c3*s2*s4)*(cx4*(c2*c4 + c3*s2*s4) - cy4*(c2*s4 - c3*c4*s2)) + 2*s2*s3*(cz4*(c2*s4 - c3*c4*s2) - cx4*s2*s3) + 2*c2*c3*c4*d3*s2) - m4*s3*(2*(c2*s4 - c3*c4*s2)*(cx4*(c2*c4 + c3*s2*s4) - cy4*(c2*s4 - c3*c4*s2)) + c4*(2*d3*c3^2*s2^2 + 2*d3*s2^2*s3^2) + 2*s2*s3*(cz4*(c2*c4 + c3*s2*s4) - cy4*s2*s3) - 2*c2*c3*d3*s2*s4)) - 2*c2*(Ixx3*c3*s2 - Ixz3*c2 + Ixy3*s2*s3) + cx3*m3*(2*c3*s2*(c2*cx3 - c3*cz3*s2) - 2*s2*s3*(c2*cy3 + cz3*s2*s3)) + cz3*m3*(2*c2*(c2*cx3 - c3*cz3*s2) + 2*s2*s3*(c3*cy3*s2 + cx3*s2*s3)) + 2*c3*s2*(Izz3*c2 - Ixz3*c3*s2 + Iyz3*s2*s3) - cx4*m4*(2*(c2*s4 - c3*c4*s2)*(cx4*(c2*c4 + c3*s2*s4) - cy4*(c2*s4 - c3*c4*s2)) + c4*(2*d3*c3^2*s2^2 + 2*d3*s2^2*s3^2) + 2*s2*s3*(cz4*(c2*c4 + c3*s2*s4) - cy4*s2*s3) - 2*c2*c3*d3*s2*s4) + cy4*m4*(s4*(2*d3*c3^2*s2^2 + 2*d3*s2^2*s3^2) - 2*(c2*c4 + c3*s2*s4)*(cx4*(c2*c4 + c3*s2*s4) - cy4*(c2*s4 - c3*c4*s2)) + 2*s2*s3*(cz4*(c2*s4 - c3*c4*s2) - cx4*s2*s3) + 2*c2*c3*c4*d3*s2)) + 2*c2*cy2*m2*(c2*cx2 - cy2*s2) + 2*cx2*m2*s2*(c2*cx2 - cy2*s2)))/2 - td2*td4*(s2*(s3*(2*Ixz4*c3 - Ixx4*c4*s3 + Iyy4*c4*s3 + Izz4*c4*s3 - 2*Ixy4*s3*s4 + cx4*m4*(2*c4*cx4*s3 - 2*cy4*s3*s4) + 2*c3*cx4*cz4*m4) + c3*(2*Iyz4*c3 + 2*Ixy4*c4*s3 - Ixx4*s3*s4 + Iyy4*s3*s4 - Izz4*s3*s4 + cy4*m4*(2*c4*cx4*s3 - 2*cy4*s3*s4) + 2*c3*cy4*cz4*m4) - d3*m4*(2*c4*cx4*s3 - 2*cy4*s3*s4)) - c2*d3*(2*c3^2*cx4*m4 - 2*c3*cy4*m4*s3)) - td1*td3*(c2*(2*Ixz3*c2 - (c2*c4 + c3*s2*s4)*(Ixy4*c4 - Ixx4*s4) - (c2*s4 - c3*c4*s2)*(Iyy4*c4 - Ixy4*s4) + d3*(c3*m4*(c4*(cx4*(c2*c4 + c3*s2*s4) - cy4*(c2*s4 - c3*c4*s2)) + (c2*c4 + c3*s2*s4)*(c4*cx4 - cy4*s4) - c3*cy4*s2 - 2*cz4*s2*s3*s4) + m4*s3*(s4*(cx4*(c2*c4 + c3*s2*s4) - cy4*(c2*s4 - c3*c4*s2)) + (c2*s4 - c3*c4*s2)*(c4*cx4 - cy4*s4) - c3*cx4*s2 + 2*c4*cz4*s2*s3)) - c4*(Ixy4*(c2*c4 + c3*s2*s4) - Ixx4*(c2*s4 - c3*c4*s2) + Ixz4*s2*s3) + s4*(Ixy4*(c2*s4 - c3*c4*s2) - Iyy4*(c2*c4 + c3*s2*s4) + Iyz4*s2*s3) - Ixx3*c3*s2 + Iyy3*c3*s2 + Izz3*c3*s2 + Izz4*c3*s2 - cx4*m4*(s4*(cx4*(c2*c4 + c3*s2*s4) - cy4*(c2*s4 - c3*c4*s2)) + (c2*s4 - c3*c4*s2)*(c4*cx4 - cy4*s4) - c3*cx4*s2 + 2*c4*cz4*s2*s3) - cy4*m4*(c4*(cx4*(c2*c4 + c3*s2*s4) - cy4*(c2*s4 - c3*c4*s2)) + (c2*c4 + c3*s2*s4)*(c4*cx4 - cy4*s4) - c3*cy4*s2 - 2*cz4*s2*s3*s4) - 2*Ixy3*s2*s3 + cx3*m3*(2*c3*cx3*s2 - 2*cy3*s2*s3) + Iyz4*s2*s3*s4 - Ixz4*c4*s2*s3 + 2*c2*cx3*cz3*m3) - s2*(2*Iyz3*c2 - c3*((c2*c4 + c3*s2*s4)*(Iyz4*c4 + Ixz4*s4) + c4*(Ixz4*(c2*s4 - c3*c4*s2) + Iyz4*(c2*c4 + c3*s2*s4) - Izz4*s2*s3) - Ixz4*c3*s2 + cz4*m4*(s4*(cx4*(c2*c4 + c3*s2*s4) - cy4*(c2*s4 - c3*c4*s2)) + (c2*s4 - c3*c4*s2)*(c4*cx4 - cy4*s4) - c3*cx4*s2 + 2*c4*cz4*s2*s3) + s2*s3*(Iyy4*c4 - Ixy4*s4) + cy4*m4*(c4*(cz4*(c2*c4 + c3*s2*s4) - cy4*s2*s3) + s4*(cz4*(c2*s4 - c3*c4*s2) - cx4*s2*s3) + c4*cz4*(c2*c4 + c3*s2*s4) + cz4*s4*(c2*s4 - c3*c4*s2) + c4*cy4*s2*s3 + cx4*s2*s3*s4) + Ixy4*s2*s3*s4 + Ixx4*c4*s2*s3) - s3*((c2*s4 - c3*c4*s2)*(Iyz4*c4 + Ixz4*s4) + s4*(Ixz4*(c2*s4 - c3*c4*s2) + Iyz4*(c2*c4 + c3*s2*s4) - Izz4*s2*s3) + Iyz4*c3*s2 - cz4*m4*(c4*(cx4*(c2*c4 + c3*s2*s4) - cy4*(c2*s4 - c3*c4*s2)) + (c2*c4 + c3*s2*s4)*(c4*cx4 - cy4*s4) - c3*cy4*s2 - 2*cz4*s2*s3*s4) - s2*s3*(Ixy4*c4 - Ixx4*s4) + cx4*m4*(c4*(cz4*(c2*c4 + c3*s2*s4) - cy4*s2*s3) + s4*(cz4*(c2*s4 - c3*c4*s2) - cx4*s2*s3) + c4*cz4*(c2*c4 + c3*s2*s4) + cz4*s4*(c2*s4 - c3*c4*s2) + c4*cy4*s2*s3 + cx4*s2*s3*s4) + Iyy4*s2*s3*s4 + Ixy4*c4*s2*s3) + 2*Ixy3*c3*s2 - Ixx3*s2*s3 + Iyy3*s2*s3 - Izz3*s2*s3 + cy3*m3*(2*c3*cx3*s2 - 2*cy3*s2*s3) + d3*m4*(c4*(cz4*(c2*c4 + c3*s2*s4) - cy4*s2*s3) + s4*(cz4*(c2*s4 - c3*c4*s2) - cx4*s2*s3) + c4*cz4*(c2*c4 + c3*s2*s4) + cz4*s4*(c2*s4 - c3*c4*s2) + c4*cy4*s2*s3 + cx4*s2*s3*s4) + 2*c2*cy3*cz3*m3)) - td1*td4*(s2*(s3*(2*Ixy4*(c2*c4 + c3*s2*s4) - Ixx4*(c2*s4 - c3*c4*s2) + Iyy4*(c2*s4 - c3*c4*s2) + Izz4*(c2*s4 - c3*c4*s2) + cx4*m4*(2*cx4*(c2*s4 - c3*c4*s2) + 2*cy4*(c2*c4 + c3*s2*s4)) + 2*Ixz4*s2*s3 + 2*cx4*cz4*m4*s2*s3) + c3*(Ixx4*(c2*c4 + c3*s2*s4) + 2*Ixy4*(c2*s4 - c3*c4*s2) - Iyy4*(c2*c4 + c3*s2*s4) + Izz4*(c2*c4 + c3*s2*s4) + cy4*m4*(2*cx4*(c2*s4 - c3*c4*s2) + 2*cy4*(c2*c4 + c3*s2*s4)) + 2*Iyz4*s2*s3 + 2*cy4*cz4*m4*s2*s3) - d3*m4*(2*cx4*(c2*s4 - c3*c4*s2) + 2*cy4*(c2*c4 + c3*s2*s4))) + c2*d3*(2*cy4*m4*s2*s3^2 - 2*c3*cx4*m4*s2*s3)) - td2*td3*(s2*(Ixx3*c3 - Iyy3*c3 + Izz3*c3 + 2*Ixy3*s3 + c3*(Ixz4*s3 - c4*(Izz4*c3 - Ixz4*c4*s3 + Iyz4*s3*s4) + c3*(Iyy4*c4 - Ixy4*s4) + Ixx4*c3*c4 + Ixy4*c3*s4 - cy4*m4*(s4*(c3*cx4 - c4*cz4*s3) + c4*(c3*cy4 + cz4*s3*s4) - c3*c4*cy4 - c3*cx4*s4) + cz4*m4*(cx4*s3 - s4*(c4*cy4*s3 + cx4*s3*s4) + 2*c3*c4*cz4 + c4*s3*(c4*cx4 - cy4*s4)) - s3*s4*(Iyz4*c4 + Ixz4*s4)) - s3*(Iyz4*s3 + c3*(Ixy4*c4 - Ixx4*s4) + s4*(Izz4*c3 - Ixz4*c4*s3 + Iyz4*s3*s4) - Ixy4*c3*c4 - Iyy4*c3*s4 + cx4*m4*(s4*(c3*cx4 - c4*cz4*s3) + c4*(c3*cy4 + cz4*s3*s4) - c3*c4*cy4 - c3*cx4*s4) - c4*s3*(Iyz4*c4 + Ixz4*s4) - cz4*m4*(c4*(c4*cy4*s3 + cx4*s3*s4) - cy4*s3 + s3*s4*(c4*cx4 - cy4*s4) + 2*c3*cz4*s4)) + d3*m4*(s4*(c3*cx4 - c4*cz4*s3) + c4*(c3*cy4 + cz4*s3*s4) - c3*c4*cy4 - c3*cx4*s4) + cy3*m3*(2*c3*cy3 + 2*cx3*s3)) - c2*(2*Ixy3*c3 - Ixx3*s3 + Iyy3*s3 + Izz3*s3 + Izz4*s3 - c4*(Ixx4*c4*s3 - Ixz4*c3 + Ixy4*s3*s4) - s4*(Iyz4*c3 + Ixy4*c4*s3 + Iyy4*s3*s4) - d3*(m4*s3*(cx4*s3 - s4*(c4*cy4*s3 + cx4*s3*s4) + 2*c3*c4*cz4 + c4*s3*(c4*cx4 - cy4*s4)) - c3*m4*(c4*(c4*cy4*s3 + cx4*s3*s4) - cy4*s3 + s3*s4*(c4*cx4 - cy4*s4) + 2*c3*cz4*s4)) + Ixz4*c3*c4 - Iyz4*c3*s4 + cx4*m4*(cx4*s3 - s4*(c4*cy4*s3 + cx4*s3*s4) + 2*c3*c4*cz4 + c4*s3*(c4*cx4 - cy4*s4)) + c4*s3*(Iyy4*c4 - Ixy4*s4) - cy4*m4*(c4*(c4*cy4*s3 + cx4*s3*s4) - cy4*s3 + s3*s4*(c4*cx4 - cy4*s4) + 2*c3*cz4*s4) - s3*s4*(Ixy4*c4 - Ixx4*s4) + cx3*m3*(2*c3*cy3 + 2*cx3*s3))) - td1*td2*(c2*((c2*c4 + c3*s2*s4)*(Ixx4*c4*s3 - Ixz4*c3 + Ixy4*s3*s4) + (c2*s4 - c3*c4*s2)*(Iyz4*c3 + Ixy4*c4*s3 + Iyy4*s3*s4) - d3*(m4*s3*((c2*s4 - c3*c4*s2)*(c4*cy4*s3 + cx4*s3*s4) - c3*(cz4*(c2*c4 + c3*s2*s4) - cy4*s2*s3) + cz4*(s2*s4 + c2*c3*c4) + s2*s3*(c3*cy4 + cz4*s3*s4) - c4*s3*(cx4*(c2*c4 + c3*s2*s4) - cy4*(c2*s4 - c3*c4*s2)) + c2*cx4*s3 - 2*c2*d3*s3*s4) + c3*m4*((c2*c4 + c3*s2*s4)*(c4*cy4*s3 + cx4*s3*s4) + c3*(cz4*(c2*s4 - c3*c4*s2) - cx4*s2*s3) + cz4*(c4*s2 - c2*c3*s4) - s2*s3*(c3*cx4 - c4*cz4*s3) + s3*s4*(cx4*(c2*c4 + c3*s2*s4) - cy4*(c2*s4 - c3*c4*s2)) + c2*cy4*s3 - 2*c2*c4*d3*s3)) - Iyz3*s2 - c2*(Ixy3*c3 - Ixx3*s3) - s3*(Izz3*c2 - Ixz3*c3*s2 + Iyz3*s2*s3) + Ixz4*(s2*s4 + c2*c3*c4) + Iyz4*(c4*s2 - c2*c3*s4) + Ixy3*c2*c3 + Iyy3*c2*s3 + Izz4*c2*s3 - cx3*m3*(s3*(c2*cx3 - c3*cz3*s2) + c3*(c2*cy3 + cz3*s2*s3) - c2*c3*cy3 - c2*cx3*s3) + c3*s2*(Iyz3*c3 + Ixz3*s3) + cz3*m3*(c3*(c3*cy3*s2 + cx3*s2*s3) - cy3*s2 + s2*s3*(c3*cx3 - cy3*s3) + 2*c2*cz3*s3) + c4*s3*(Ixy4*(c2*s4 - c3*c4*s2) - Iyy4*(c2*c4 + c3*s2*s4) + Iyz4*s2*s3) + s3*s4*(Ixy4*(c2*c4 + c3*s2*s4) - Ixx4*(c2*s4 - c3*c4*s2) + Ixz4*s2*s3) + cy4*m4*((c2*c4 + c3*s2*s4)*(c4*cy4*s3 + cx4*s3*s4) + c3*(cz4*(c2*s4 - c3*c4*s2) - cx4*s2*s3) + cz4*(c4*s2 - c2*c3*s4) - s2*s3*(c3*cx4 - c4*cz4*s3) + s3*s4*(cx4*(c2*c4 + c3*s2*s4) - cy4*(c2*s4 - c3*c4*s2)) + c2*cy4*s3 - 2*c2*c4*d3*s3) + cx4*m4*((c2*s4 - c3*c4*s2)*(c4*cy4*s3 + cx4*s3*s4) - c3*(cz4*(c2*c4 + c3*s2*s4) - cy4*s2*s3) + cz4*(s2*s4 + c2*c3*c4) + s2*s3*(c3*cy4 + cz4*s3*s4) - c4*s3*(cx4*(c2*c4 + c3*s2*s4) - cy4*(c2*s4 - c3*c4*s2)) + c2*cx4*s3 - 2*c2*d3*s3*s4)) - s2*(c3*((c2*c4 + c3*s2*s4)*(Izz4*c3 - Ixz4*c4*s3 + Iyz4*s3*s4) + c3*(Ixy4*(c2*s4 - c3*c4*s2) - Iyy4*(c2*c4 + c3*s2*s4) + Iyz4*s2*s3) + Ixx4*(s2*s4 + c2*c3*c4) - Ixy4*(c4*s2 - c2*c3*s4) + Ixz4*c2*s3 + s2*s3*(Iyz4*c3 + Ixy4*c4*s3 + Iyy4*s3*s4) + cy4*m4*((c3*cx4 - c4*cz4*s3)*(c2*s4 - c3*c4*s2) + (c2*c4 + c3*s2*s4)*(c3*cy4 + cz4*s3*s4) - cx4*(c4*s2 - c2*c3*s4) + cy4*(s2*s4 + c2*c3*c4) - c4*s3*(cz4*(c2*s4 - c3*c4*s2) - cx4*s2*s3) + s3*s4*(cz4*(c2*c4 + c3*s2*s4) - cy4*s2*s3) - 2*c2*c3*d3) + s3*s4*(Ixz4*(c2*s4 - c3*c4*s2) + Iyz4*(c2*c4 + c3*s2*s4) - Izz4*s2*s3) + cz4*m4*((c2*s4 - c3*c4*s2)*(c4*cy4*s3 + cx4*s3*s4) - c3*(cz4*(c2*c4 + c3*s2*s4) - cy4*s2*s3) + cz4*(s2*s4 + c2*c3*c4) + s2*s3*(c3*cy4 + cz4*s3*s4) - c4*s3*(cx4*(c2*c4 + c3*s2*s4) - cy4*(c2*s4 - c3*c4*s2)) + c2*cx4*s3 - 2*c2*d3*s3*s4)) - s3*(Iyy4*(c4*s2 - c2*c3*s4) - c3*(Ixy4*(c2*c4 + c3*s2*s4) - Ixx4*(c2*s4 - c3*c4*s2) + Ixz4*s2*s3) - Ixy4*(s2*s4 + c2*c3*c4) - (c2*s4 - c3*c4*s2)*(Izz4*c3 - Ixz4*c4*s3 + Iyz4*s3*s4) + Iyz4*c2*s3 + s2*s3*(Ixx4*c4*s3 - Ixz4*c3 + Ixy4*s3*s4) - cx4*m4*((c3*cx4 - c4*cz4*s3)*(c2*s4 - c3*c4*s2) + (c2*c4 + c3*s2*s4)*(c3*cy4 + cz4*s3*s4) - cx4*(c4*s2 - c2*c3*s4) + cy4*(s2*s4 + c2*c3*c4) - c4*s3*(cz4*(c2*s4 - c3*c4*s2) - cx4*s2*s3) + s3*s4*(cz4*(c2*c4 + c3*s2*s4) - cy4*s2*s3) - 2*c2*c3*d3) + c4*s3*(Ixz4*(c2*s4 - c3*c4*s2) + Iyz4*(c2*c4 + c3*s2*s4) - Izz4*s2*s3) + cz4*m4*((c2*c4 + c3*s2*s4)*(c4*cy4*s3 + cx4*s3*s4) + c3*(cz4*(c2*s4 - c3*c4*s2) - cx4*s2*s3) + cz4*(c4*s2 - c2*c3*s4) - s2*s3*(c3*cx4 - c4*cz4*s3) + s3*s4*(cx4*(c2*c4 + c3*s2*s4) - cy4*(c2*s4 - c3*c4*s2)) + c2*cy4*s3 - 2*c2*c4*d3*s3)) + Ixz3*s2 - c3*(Izz3*c2 - Ixz3*c3*s2 + Iyz3*s2*s3) + c2*(Iyy3*c3 - Ixy3*s3) + Ixx3*c2*c3 + Ixy3*c2*s3 - cy3*m3*(s3*(c2*cx3 - c3*cz3*s2) + c3*(c2*cy3 + cz3*s2*s3) - c2*c3*cy3 - c2*cx3*s3) + cz3*m3*(cx3*s2 - s3*(c3*cy3*s2 + cx3*s2*s3) + 2*c2*c3*cz3 + c3*s2*(c3*cx3 - cy3*s3)) - d3*m4*((c3*cx4 - c4*cz4*s3)*(c2*s4 - c3*c4*s2) + (c2*c4 + c3*s2*s4)*(c3*cy4 + cz4*s3*s4) - cx4*(c4*s2 - c2*c3*s4) + cy4*(s2*s4 + c2*c3*c4) - c4*s3*(cz4*(c2*s4 - c3*c4*s2) - cx4*s2*s3) + s3*s4*(cz4*(c2*c4 + c3*s2*s4) - cy4*s2*s3) - 2*c2*c3*d3) - s2*s3*(Iyz3*c3 + Ixz3*s3))) - s2*td3*td4*(c3*(Ixx4*c4 - Iyy4*c4 + Izz4*c4 + 2*Ixy4*s4 + cy4*m4*(2*c4*cy4 + 2*cx4*s4)) + s3*(2*Ixy4*c4 - Ixx4*s4 + Iyy4*s4 + Izz4*s4 + cx4*m4*(2*c4*cy4 + 2*cx4*s4)) - d3*m4*(2*c4*cy4 + 2*cx4*s4));
corio3 = (td2^2*(c3*(cx4*m4*(2*c4*s3*(c3*cx4 - c4*cz4*s3) - 2*s3*s4*(c3*cy4 + cz4*s3*s4)) - 2*c3*(Ixx4*c4*s3 - Ixz4*c3 + Ixy4*s3*s4) + cz4*m4*(2*c3*(c3*cx4 - c4*cz4*s3) - s4*(2*d3*c3^2 + 2*d3*s3^2) + 2*s3*s4*(c4*cy4*s3 + cx4*s3*s4)) + 2*c4*s3*(Izz4*c3 - Ixz4*c4*s3 + Iyz4*s3*s4)) - s3*(2*c3*(Iyz4*c3 + Ixy4*c4*s3 + Iyy4*s3*s4) + cy4*m4*(2*c4*s3*(c3*cx4 - c4*cz4*s3) - 2*s3*s4*(c3*cy4 + cz4*s3*s4)) + cz4*m4*(2*c3*(c3*cy4 + cz4*s3*s4) - c4*(2*d3*c3^2 + 2*d3*s3^2) + 2*c4*s3*(c4*cy4*s3 + cx4*s3*s4)) - 2*s3*s4*(Izz4*c3 - Ixz4*c4*s3 + Iyz4*s3*s4)) + 2*c3*(Ixy3*c3 - Ixx3*s3) + 2*s3*(Iyy3*c3 - Ixy3*s3) + 2*c3*cy3*m3*(c3*cx3 - cy3*s3) + 2*cx3*m3*s3*(c3*cx3 - cy3*s3)))/2 - (td1^2*(c3*(2*(c2*s4 - c3*c4*s2)*(Ixz4*(c2*s4 - c3*c4*s2) + Iyz4*(c2*c4 + c3*s2*s4) - Izz4*s2*s3) + cx4*m4*(2*(c2*s4 - c3*c4*s2)*(cz4*(c2*s4 - c3*c4*s2) - cx4*s2*s3) + 2*(c2*c4 + c3*s2*s4)*(cz4*(c2*c4 + c3*s2*s4) - cy4*s2*s3) + 2*c2*d3*s2*s3) - 2*s2*s3*(Ixy4*(c2*c4 + c3*s2*s4) - Ixx4*(c2*s4 - c3*c4*s2) + Ixz4*s2*s3) + cz4*m4*(s4*(2*d3*c3^2*s2^2 + 2*d3*s2^2*s3^2) - 2*(c2*c4 + c3*s2*s4)*(cx4*(c2*c4 + c3*s2*s4) - cy4*(c2*s4 - c3*c4*s2)) + 2*s2*s3*(cz4*(c2*s4 - c3*c4*s2) - cx4*s2*s3) + 2*c2*c3*c4*d3*s2)) - s3*(2*(c2*c4 + c3*s2*s4)*(Ixz4*(c2*s4 - c3*c4*s2) + Iyz4*(c2*c4 + c3*s2*s4) - Izz4*s2*s3) + cy4*m4*(2*(c2*s4 - c3*c4*s2)*(cz4*(c2*s4 - c3*c4*s2) - cx4*s2*s3) + 2*(c2*c4 + c3*s2*s4)*(cz4*(c2*c4 + c3*s2*s4) - cy4*s2*s3) + 2*c2*d3*s2*s3) - 2*s2*s3*(Ixy4*(c2*s4 - c3*c4*s2) - Iyy4*(c2*c4 + c3*s2*s4) + Iyz4*s2*s3) + cz4*m4*(2*(c2*s4 - c3*c4*s2)*(cx4*(c2*c4 + c3*s2*s4) - cy4*(c2*s4 - c3*c4*s2)) + c4*(2*d3*c3^2*s2^2 + 2*d3*s2^2*s3^2) + 2*s2*s3*(cz4*(c2*c4 + c3*s2*s4) - cy4*s2*s3) - 2*c2*c3*d3*s2*s4)) + cx3*m3*(2*c2*(c2*cy3 + cz3*s2*s3) + 2*c3*s2*(c3*cy3*s2 + cx3*s2*s3)) - cy3*m3*(2*c2*(c2*cx3 - c3*cz3*s2) + 2*s2*s3*(c3*cy3*s2 + cx3*s2*s3)) + 2*c3*s2*(Iyz3*c2 + Ixy3*c3*s2 + Iyy3*s2*s3) - 2*s2*s3*(Ixx3*c3*s2 - Ixz3*c2 + Ixy3*s2*s3)))/2 + (td4^2*(c3*(2*Ixz4 + 2*cx4*cz4*m4) - s3*(2*Iyz4 + 2*cy4*cz4*m4)))/2 - (td3^2*(c3*(2*s4*(Iyz4*c4 + Ixz4*s4) + cx4*m4*(2*cz4*c4^2 + 2*cz4*s4^2) - 2*c4*cz4*m4*(c4*cx4 - cy4*s4)) - s3*(2*c4*(Iyz4*c4 + Ixz4*s4) + cy4*m4*(2*cz4*c4^2 + 2*cz4*s4^2) + 2*cz4*m4*s4*(c4*cx4 - cy4*s4))))/2 - td1*td2*(Izz3*s2 + s3*((c2*c4 + c3*s2*s4)*(Izz4*c3 - Ixz4*c4*s3 + Iyz4*s3*s4) + c3*(Ixy4*(c2*s4 - c3*c4*s2) - Iyy4*(c2*c4 + c3*s2*s4) + Iyz4*s2*s3) + Ixx4*(s2*s4 + c2*c3*c4) - Ixy4*(c4*s2 - c2*c3*s4) + Ixz4*c2*s3 + s2*s3*(Iyz4*c3 + Ixy4*c4*s3 + Iyy4*s3*s4) + cy4*m4*((c3*cx4 - c4*cz4*s3)*(c2*s4 - c3*c4*s2) + (c2*c4 + c3*s2*s4)*(c3*cy4 + cz4*s3*s4) - cx4*(c4*s2 - c2*c3*s4) + cy4*(s2*s4 + c2*c3*c4) - c4*s3*(cz4*(c2*s4 - c3*c4*s2) - cx4*s2*s3) + s3*s4*(cz4*(c2*c4 + c3*s2*s4) - cy4*s2*s3) - 2*c2*c3*d3) + s3*s4*(Ixz4*(c2*s4 - c3*c4*s2) + Iyz4*(c2*c4 + c3*s2*s4) - Izz4*s2*s3) + cz4*m4*((c2*s4 - c3*c4*s2)*(c4*cy4*s3 + cx4*s3*s4) - c3*(cz4*(c2*c4 + c3*s2*s4) - cy4*s2*s3) + cz4*(s2*s4 + c2*c3*c4) + s2*s3*(c3*cy4 + cz4*s3*s4) - c4*s3*(cx4*(c2*c4 + c3*s2*s4) - cy4*(c2*s4 - c3*c4*s2)) + c2*cx4*s3 - 2*c2*d3*s3*s4)) - c3*(Ixx3*c3*s2 - Ixz3*c2 + Ixy3*s2*s3) - s3*(Iyz3*c2 + Ixy3*c3*s2 + Iyy3*s2*s3) + c3*(Iyy4*(c4*s2 - c2*c3*s4) - c3*(Ixy4*(c2*c4 + c3*s2*s4) - Ixx4*(c2*s4 - c3*c4*s2) + Ixz4*s2*s3) - Ixy4*(s2*s4 + c2*c3*c4) - (c2*s4 - c3*c4*s2)*(Izz4*c3 - Ixz4*c4*s3 + Iyz4*s3*s4) + Iyz4*c2*s3 + s2*s3*(Ixx4*c4*s3 - Ixz4*c3 + Ixy4*s3*s4) - cx4*m4*((c3*cx4 - c4*cz4*s3)*(c2*s4 - c3*c4*s2) + (c2*c4 + c3*s2*s4)*(c3*cy4 + cz4*s3*s4) - cx4*(c4*s2 - c2*c3*s4) + cy4*(s2*s4 + c2*c3*c4) - c4*s3*(cz4*(c2*s4 - c3*c4*s2) - cx4*s2*s3) + s3*s4*(cz4*(c2*c4 + c3*s2*s4) - cy4*s2*s3) - 2*c2*c3*d3) + c4*s3*(Ixz4*(c2*s4 - c3*c4*s2) + Iyz4*(c2*c4 + c3*s2*s4) - Izz4*s2*s3) + cz4*m4*((c2*c4 + c3*s2*s4)*(c4*cy4*s3 + cx4*s3*s4) + c3*(cz4*(c2*s4 - c3*c4*s2) - cx4*s2*s3) + cz4*(c4*s2 - c2*c3*s4) - s2*s3*(c3*cx4 - c4*cz4*s3) + s3*s4*(cx4*(c2*c4 + c3*s2*s4) - cy4*(c2*s4 - c3*c4*s2)) + c2*cy4*s3 - 2*c2*c4*d3*s3)) + Ixz3*c2*c3 - Iyz3*c2*s3 + cx3*m3*(cx3*s2 - s3*(c3*cy3*s2 + cx3*s2*s3) + 2*c2*c3*cz3 + c3*s2*(c3*cx3 - cy3*s3)) + c3*s2*(Iyy3*c3 - Ixy3*s3) - cy3*m3*(c3*(c3*cy3*s2 + cx3*s2*s3) - cy3*s2 + s2*s3*(c3*cx3 - cy3*s3) + 2*c2*cz3*s3) - s2*s3*(Ixy3*c3 - Ixx3*s3)) + td2*td3*(s3*(Ixz4*s3 - c4*(Izz4*c3 - Ixz4*c4*s3 + Iyz4*s3*s4) + c3*(Iyy4*c4 - Ixy4*s4) + Ixx4*c3*c4 + Ixy4*c3*s4 - cy4*m4*(s4*(c3*cx4 - c4*cz4*s3) + c4*(c3*cy4 + cz4*s3*s4) - c3*c4*cy4 - c3*cx4*s4) + cz4*m4*(cx4*s3 - s4*(c4*cy4*s3 + cx4*s3*s4) + 2*c3*c4*cz4 + c4*s3*(c4*cx4 - cy4*s4)) - s3*s4*(Iyz4*c4 + Ixz4*s4)) + c3*(Iyz4*s3 + c3*(Ixy4*c4 - Ixx4*s4) + s4*(Izz4*c3 - Ixz4*c4*s3 + Iyz4*s3*s4) - Ixy4*c3*c4 - Iyy4*c3*s4 + cx4*m4*(s4*(c3*cx4 - c4*cz4*s3) + c4*(c3*cy4 + cz4*s3*s4) - c3*c4*cy4 - c3*cx4*s4) - c4*s3*(Iyz4*c4 + Ixz4*s4) - cz4*m4*(c4*(c4*cy4*s3 + cx4*s3*s4) - cy4*s3 + s3*s4*(c4*cx4 - cy4*s4) + 2*c3*cz4*s4))) + td1*td3*(s3*((c2*c4 + c3*s2*s4)*(Iyz4*c4 + Ixz4*s4) + c4*(Ixz4*(c2*s4 - c3*c4*s2) + Iyz4*(c2*c4 + c3*s2*s4) - Izz4*s2*s3) - Ixz4*c3*s2 + cz4*m4*(s4*(cx4*(c2*c4 + c3*s2*s4) - cy4*(c2*s4 - c3*c4*s2)) + (c2*s4 - c3*c4*s2)*(c4*cx4 - cy4*s4) - c3*cx4*s2 + 2*c4*cz4*s2*s3) + s2*s3*(Iyy4*c4 - Ixy4*s4) + cy4*m4*(c4*(cz4*(c2*c4 + c3*s2*s4) - cy4*s2*s3) + s4*(cz4*(c2*s4 - c3*c4*s2) - cx4*s2*s3) + c4*cz4*(c2*c4 + c3*s2*s4) + cz4*s4*(c2*s4 - c3*c4*s2) + c4*cy4*s2*s3 + cx4*s2*s3*s4) + Ixy4*s2*s3*s4 + Ixx4*c4*s2*s3) - c3*((c2*s4 - c3*c4*s2)*(Iyz4*c4 + Ixz4*s4) + s4*(Ixz4*(c2*s4 - c3*c4*s2) + Iyz4*(c2*c4 + c3*s2*s4) - Izz4*s2*s3) + Iyz4*c3*s2 - cz4*m4*(c4*(cx4*(c2*c4 + c3*s2*s4) - cy4*(c2*s4 - c3*c4*s2)) + (c2*c4 + c3*s2*s4)*(c4*cx4 - cy4*s4) - c3*cy4*s2 - 2*cz4*s2*s3*s4) - s2*s3*(Ixy4*c4 - Ixx4*s4) + cx4*m4*(c4*(cz4*(c2*c4 + c3*s2*s4) - cy4*s2*s3) + s4*(cz4*(c2*s4 - c3*c4*s2) - cx4*s2*s3) + c4*cz4*(c2*c4 + c3*s2*s4) + cz4*s4*(c2*s4 - c3*c4*s2) + c4*cy4*s2*s3 + cx4*s2*s3*s4) + Iyy4*s2*s3*s4 + Ixy4*c4*s2*s3)) + td3*td4*(s3*(Ixx4*c4 - Iyy4*c4 + Izz4*c4 + 2*Ixy4*s4 + cy4*m4*(2*c4*cy4 + 2*cx4*s4)) - c3*(2*Ixy4*c4 - Ixx4*s4 + Iyy4*s4 + Izz4*s4 + cx4*m4*(2*c4*cy4 + 2*cx4*s4))) + td1*td4*(s3*(Ixx4*(c2*c4 + c3*s2*s4) + 2*Ixy4*(c2*s4 - c3*c4*s2) - Iyy4*(c2*c4 + c3*s2*s4) + Izz4*(c2*c4 + c3*s2*s4) + cy4*m4*(2*cx4*(c2*s4 - c3*c4*s2) + 2*cy4*(c2*c4 + c3*s2*s4)) + 2*Iyz4*s2*s3 + 2*cy4*cz4*m4*s2*s3) - c3*(2*Ixy4*(c2*c4 + c3*s2*s4) - Ixx4*(c2*s4 - c3*c4*s2) + Iyy4*(c2*s4 - c3*c4*s2) + Izz4*(c2*s4 - c3*c4*s2) + cx4*m4*(2*cx4*(c2*s4 - c3*c4*s2) + 2*cy4*(c2*c4 + c3*s2*s4)) + 2*Ixz4*s2*s3 + 2*cx4*cz4*m4*s2*s3)) - td2*td4*(c3*(2*Ixz4*c3 - Ixx4*c4*s3 + Iyy4*c4*s3 + Izz4*c4*s3 - 2*Ixy4*s3*s4 + cx4*m4*(2*c4*cx4*s3 - 2*cy4*s3*s4) + 2*c3*cx4*cz4*m4) - s3*(2*Iyz4*c3 + 2*Ixy4*c4*s3 - Ixx4*s3*s4 + Iyy4*s3*s4 - Izz4*s3*s4 + cy4*m4*(2*c4*cx4*s3 - 2*cy4*s3*s4) + 2*c3*cy4*cz4*m4));
corio4 = (td1^2*(2*(c2*c4 + c3*s2*s4)*(Ixy4*(c2*c4 + c3*s2*s4) - Ixx4*(c2*s4 - c3*c4*s2) + Ixz4*s2*s3) - 2*(c2*s4 - c3*c4*s2)*(Ixy4*(c2*s4 - c3*c4*s2) - Iyy4*(c2*c4 + c3*s2*s4) + Iyz4*s2*s3) + cx4*m4*(2*(c2*s4 - c3*c4*s2)*(cx4*(c2*c4 + c3*s2*s4) - cy4*(c2*s4 - c3*c4*s2)) + c4*(2*d3*c3^2*s2^2 + 2*d3*s2^2*s3^2) + 2*s2*s3*(cz4*(c2*c4 + c3*s2*s4) - cy4*s2*s3) - 2*c2*c3*d3*s2*s4) - cy4*m4*(s4*(2*d3*c3^2*s2^2 + 2*d3*s2^2*s3^2) - 2*(c2*c4 + c3*s2*s4)*(cx4*(c2*c4 + c3*s2*s4) - cy4*(c2*s4 - c3*c4*s2)) + 2*s2*s3*(cz4*(c2*s4 - c3*c4*s2) - cx4*s2*s3) + 2*c2*c3*c4*d3*s2)))/2 - (td2^2*(cx4*m4*(2*c3*(c3*cy4 + cz4*s3*s4) - c4*(2*d3*c3^2 + 2*d3*s3^2) + 2*c4*s3*(c4*cy4*s3 + cx4*s3*s4)) - cy4*m4*(2*c3*(c3*cx4 - c4*cz4*s3) - s4*(2*d3*c3^2 + 2*d3*s3^2) + 2*s3*s4*(c4*cy4*s3 + cx4*s3*s4)) + 2*c4*s3*(Iyz4*c3 + Ixy4*c4*s3 + Iyy4*s3*s4) - 2*s3*s4*(Ixx4*c4*s3 - Ixz4*c3 + Ixy4*s3*s4)))/2 + (td3^2*(2*c4*(Ixy4*c4 - Ixx4*s4) + 2*s4*(Iyy4*c4 - Ixy4*s4) + 2*c4*cy4*m4*(c4*cx4 - cy4*s4) + 2*cx4*m4*s4*(c4*cx4 - cy4*s4)))/2 + td1*td3*((c2*c4 + c3*s2*s4)*(Ixy4*c4 - Ixx4*s4) + (c2*s4 - c3*c4*s2)*(Iyy4*c4 - Ixy4*s4) + c4*(Ixy4*(c2*c4 + c3*s2*s4) - Ixx4*(c2*s4 - c3*c4*s2) + Ixz4*s2*s3) - s4*(Ixy4*(c2*s4 - c3*c4*s2) - Iyy4*(c2*c4 + c3*s2*s4) + Iyz4*s2*s3) - Izz4*c3*s2 + cx4*m4*(s4*(cx4*(c2*c4 + c3*s2*s4) - cy4*(c2*s4 - c3*c4*s2)) + (c2*s4 - c3*c4*s2)*(c4*cx4 - cy4*s4) - c3*cx4*s2 + 2*c4*cz4*s2*s3) + cy4*m4*(c4*(cx4*(c2*c4 + c3*s2*s4) - cy4*(c2*s4 - c3*c4*s2)) + (c2*c4 + c3*s2*s4)*(c4*cx4 - cy4*s4) - c3*cy4*s2 - 2*cz4*s2*s3*s4) - Iyz4*s2*s3*s4 + Ixz4*c4*s2*s3) - td2*td3*(c4*(Ixx4*c4*s3 - Ixz4*c3 + Ixy4*s3*s4) - Izz4*s3 + s4*(Iyz4*c3 + Ixy4*c4*s3 + Iyy4*s3*s4) - Ixz4*c3*c4 + Iyz4*c3*s4 - cx4*m4*(cx4*s3 - s4*(c4*cy4*s3 + cx4*s3*s4) + 2*c3*c4*cz4 + c4*s3*(c4*cx4 - cy4*s4)) - c4*s3*(Iyy4*c4 - Ixy4*s4) + cy4*m4*(c4*(c4*cy4*s3 + cx4*s3*s4) - cy4*s3 + s3*s4*(c4*cx4 - cy4*s4) + 2*c3*cz4*s4) + s3*s4*(Ixy4*c4 - Ixx4*s4)) - td1*td2*((c2*c4 + c3*s2*s4)*(Ixx4*c4*s3 - Ixz4*c3 + Ixy4*s3*s4) + (c2*s4 - c3*c4*s2)*(Iyz4*c3 + Ixy4*c4*s3 + Iyy4*s3*s4) + Ixz4*(s2*s4 + c2*c3*c4) + Iyz4*(c4*s2 - c2*c3*s4) + Izz4*c2*s3 + c4*s3*(Ixy4*(c2*s4 - c3*c4*s2) - Iyy4*(c2*c4 + c3*s2*s4) + Iyz4*s2*s3) + s3*s4*(Ixy4*(c2*c4 + c3*s2*s4) - Ixx4*(c2*s4 - c3*c4*s2) + Ixz4*s2*s3) + cy4*m4*((c2*c4 + c3*s2*s4)*(c4*cy4*s3 + cx4*s3*s4) + c3*(cz4*(c2*s4 - c3*c4*s2) - cx4*s2*s3) + cz4*(c4*s2 - c2*c3*s4) - s2*s3*(c3*cx4 - c4*cz4*s3) + s3*s4*(cx4*(c2*c4 + c3*s2*s4) - cy4*(c2*s4 - c3*c4*s2)) + c2*cy4*s3 - 2*c2*c4*d3*s3) + cx4*m4*((c2*s4 - c3*c4*s2)*(c4*cy4*s3 + cx4*s3*s4) - c3*(cz4*(c2*c4 + c3*s2*s4) - cy4*s2*s3) + cz4*(s2*s4 + c2*c3*c4) + s2*s3*(c3*cy4 + cz4*s3*s4) - c4*s3*(cx4*(c2*c4 + c3*s2*s4) - cy4*(c2*s4 - c3*c4*s2)) + c2*cx4*s3 - 2*c2*d3*s3*s4));

V = [corio1;
     corio2;
     corio3;
     corio4];
 
 %% matrix G
 
 g1 = g*(s2*(c3*(cz4*m4*(c2*c4 + c3*s2*s4) - cy4*m4*s2*s3) + s3*(cz4*m4*(c2*s4 - c3*c4*s2) - cx4*m4*s2*s3) + c2*cy3*m3 + cz3*m3*s2*s3 + d3*m4*s2*s3) - c2*(d3*(c3*m4*(c2*s4 - c3*c4*s2) - m4*s3*(c2*c4 + c3*s2*s4)) + cx4*m4*(c2*c4 + c3*s2*s4) - cy4*m4*(c2*s4 - c3*c4*s2) + c2*cx3*m3 - c3*cz3*m3*s2) + c2*cx2*m2 - cy2*m2*s2);
 g2 = g*(s2*(c3*(cz4*m4*(c2*c4 + c3*s2*s4) - cy4*m4*s2*s3) + s3*(cz4*m4*(c2*s4 - c3*c4*s2) - cx4*m4*s2*s3) + c2*cy3*m3 + cz3*m3*s2*s3 + d3*m4*s2*s3) - c2*(d3*(c3*m4*(c2*s4 - c3*c4*s2) - m4*s3*(c2*c4 + c3*s2*s4)) + cx4*m4*(c2*c4 + c3*s2*s4) - cy4*m4*(c2*s4 - c3*c4*s2) + c2*cx3*m3 - c3*cz3*m3*s2) + c2*cx2*m2 - cy2*m2*s2);
 g3 = -g*(s3*(cz4*m4*(c2*c4 + c3*s2*s4) - cy4*m4*s2*s3) - c3*(cz4*m4*(c2*s4 - c3*c4*s2) - cx4*m4*s2*s3) + c3*cy3*m3*s2 + cx3*m3*s2*s3);
 g4 = -g*(cx4*m4*(c2*c4 + c3*s2*s4) - cy4*m4*(c2*s4 - c3*c4*s2));
 
 G = [g1;
     g2;
     g3;
     g4];
 
%% out put

q_ddot = pinv(M)*(torque - V - G);
